simulink model "network_motif_controller_linear"  (R2022b)
settings: Solver=VariableStepAuto  StartTime=0.0  StopTime=120  RelTol=1e-3
settings Model: Creator=u1473578  LastModifiedBy=u1473578
settings DebuggingCC: UnconnectedInputMsg=warning  UnconnectedOutputMsg=warning  UnconnectedLineMsg=warning
settings ModelReferenceCC: EnableRefExpFcnMdlSchedulingChecks=on
settings RTWCC: DLArmComputeVersion=19.05

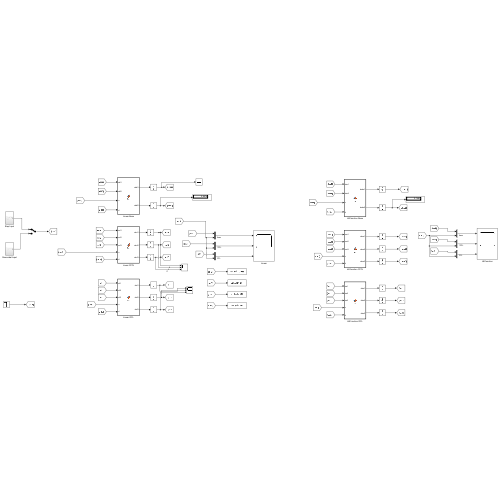
[thumbnail: Simulink's stored preview of the top-level diagram]
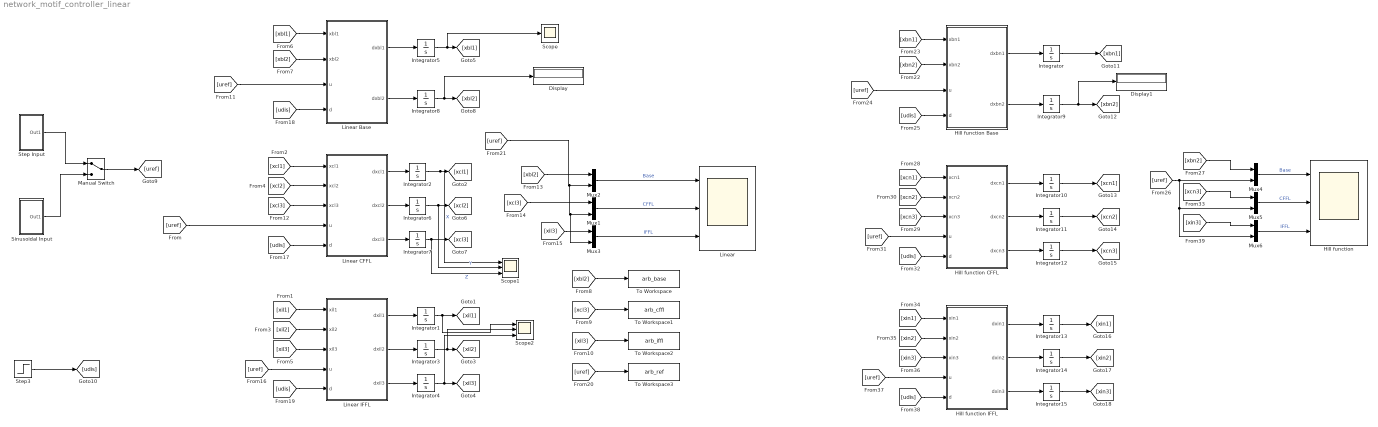
== system network_motif_controller_linear ==
  Display : Display
  Display1 : Display
  Hill function : Scope  NumInputPorts=3
  Hill function Base : MATLAB Function  TreatAsAtomicUnit=on
  Hill function CFFL : MATLAB Function  TreatAsAtomicUnit=on
  Hill function IFFL : MATLAB Function  TreatAsAtomicUnit=on
  Integrator{,1..15} (16 alike) : Integrator
  Linear : Scope  NumInputPorts=3
  Linear Base : MATLAB Function  TreatAsAtomicUnit=on
  Linear CFFL : MATLAB Function  TreatAsAtomicUnit=on
  Linear IFFL : MATLAB Function  TreatAsAtomicUnit=on
  Manual Switch : ManualSwitch
  Mux{1..6} (6 alike) : Mux  Inputs=2
  Scope : Scope
  Scope1 : Scope  NumInputPorts=3
  Scope2 : Scope  NumInputPorts=3
  Sinusoidal Input : Subsystem
  Step Input : Subsystem
  Step3 : Step  Time=60  After=-0.25*1  SampleTime=0
  To Workspace : ToWorkspace  VariableName=arb_base  SaveFormat=Timeseries  SampleTime=-1
  To Workspace1 : ToWorkspace  VariableName=arb_cffl  SaveFormat=Timeseries  SampleTime=-1
  To Workspace2 : ToWorkspace  VariableName=arb_iffl  SaveFormat=Timeseries  SampleTime=-1
  To Workspace3 : ToWorkspace  VariableName=arb_ref  SaveFormat=Timeseries  SampleTime=-1
  wires:
  Integrator2/1 -> Scope1/1, [xcl1]  "X"
  Linear CFFL/3(dxcl3) -> Integrator7/1
  [xil3] -> Mux3/1
  [xcl1] -> Linear CFFL/1(xcl1)
  Integrator7/1 -> Scope1/3, [xcl3]  "Z"
  [xcl2] -> Linear CFFL/2(xcl2)
  Mux3/1 -> Linear/3  "IFFL"
  [xcl3] -> Linear CFFL/3(xcl3)
  Linear CFFL/2(dxcl2) -> Integrator6/1
  Integrator6/1 -> Scope1/2, [xcl2]  "Y"
  Linear CFFL/1(dxcl1) -> Integrator2/1
  [xil1] -> Linear IFFL/1(xil1)
  [xil2] -> Linear IFFL/2(xil2)
  [xil3] -> Linear IFFL/3(xil3)
  Linear IFFL/1(dxil1) -> Integrator1/1
  Linear IFFL/2(dxil2) -> Integrator3/1
  Linear IFFL/3(dxil3) -> Integrator4/1
  Integrator1/1 -> Scope2/1, [xil1]
  Integrator3/1 -> Scope2/2, [xil2]
  Integrator4/1 -> Scope2/3, [xil3]
  [xcl3] -> Mux1/1
  Mux1/1 -> Linear/2  "CFFL"
  [xbl1] -> Linear Base/1(xbl1)
  [xbl2] -> Linear Base/2(xbl2)
  Linear Base/1(dxbl1) -> Integrator5/1
  Linear Base/2(dxbl2) -> Integrator8/1
  Integrator5/1 -> Scope/1, [xbl1]
  Integrator8/1 -> Display/1, [xbl2]
  Mux2/1 -> Linear/1  "Base"
  [xbl2] -> Mux2/1
  [xcl3] -> To Workspace1/1
  [xil3] -> To Workspace2/1
  [xbl2] -> To Workspace/1
  [uref] -> Linear CFFL/4(u)
  [uref] -> Linear Base/3(u)
  [uref] -> Linear IFFL/4(u)
  Step3/1 -> [udis]
  [udis] -> Linear CFFL/5(d)
  [udis] -> Linear Base/4(d)
  [udis] -> Linear IFFL/5(d)
  [uref] -> To Workspace3/1
  [uref] -> Mux3/2, Mux1/2, Mux2/2
  Hill function Base/1(dxbn1) -> Integrator/1
  Hill function Base/2(dxbn2) -> Integrator9/1
  Integrator/1 -> [xbn1]
  Integrator9/1 -> Display1/1, [xbn2]
  [xbn2] -> Hill function Base/2(xbn2)
  [xbn1] -> Hill function Base/1(xbn1)
  [uref] -> Hill function Base/3(u)
  [udis] -> Hill function Base/4(d)
  [uref] -> Mux6/2, Mux5/2, Mux4/2
  [xbn2] -> Mux4/1
  Mux4/1 -> Hill function/1  "Base"
  Hill function CFFL/1(dxcn1) -> Integrator10/1
  Hill function CFFL/2(dxcn2) -> Integrator11/1
  Hill function CFFL/3(dxcn3) -> Integrator12/1
  Integrator10/1 -> [xcn1]
  Integrator11/1 -> [xcn2]
  Integrator12/1 -> [xcn3]
  [xcn3] -> Hill function CFFL/3(xcn3)
  [xcn2] -> Hill function CFFL/2(xcn2)
  [xcn1] -> Hill function CFFL/1(xcn1)
  [uref] -> Hill function CFFL/4(u)
  [udis] -> Hill function CFFL/5(d)
  Mux5/1 -> Hill function/2  "CFFL"
  [xcn3] -> Mux5/1
  Hill function IFFL/1(dxin1) -> Integrator13/1
  Hill function IFFL/2(dxin2) -> Integrator14/1
  Hill function IFFL/3(dxin3) -> Integrator15/1
  Integrator13/1 -> [xin1]
  Integrator14/1 -> [xin2]
  Integrator15/1 -> [xin3]
  [xin1] -> Hill function IFFL/1(xin1)
  [xin2] -> Hill function IFFL/2(xin2)
  [xin3] -> Hill function IFFL/3(xin3)
  [uref] -> Hill function IFFL/4(u)
  [udis] -> Hill function IFFL/5(d)
  Mux6/1 -> Hill function/3  "IFFL"
  [xin3] -> Mux6/1
  Step Input/1(Out1) -> Manual Switch/1
  Sinusoidal Input/1(Out1) -> Manual Switch/2
  Manual Switch/1 -> [uref]

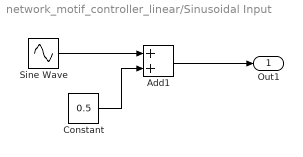
== system network_motif_controller_linear/Sinusoidal Input ==
  Add1 : Sum
  Constant : Constant  Value=0.5
  Sine Wave : Sin  Amplitude=0.5  Frequency=10/120  Phase=2800-150  SampleTime=0
  Out1 : Outport
  wires:
  Sine Wave/1 -> Add1/1
  Constant/1 -> Add1/2
  Add1/1 -> Out1/1

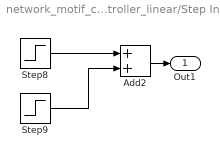
== system network_motif_controller_linear/Step Input ==
  Add2 : Sum
  Step8 : Step  Time=0  After=0  SampleTime=0
  Step9 : Step  Time=40  SampleTime=0
  Out1 : Outport
  wires:
  Step8/1 -> Add2/1
  Step9/1 -> Add2/2
  Add2/1 -> Out1/1

== matlab function network_motif_controller_linear/Linear IFFL ==
  data: xil1 input; xil2 input; xil3 input; u input; dxil1 output; dxil2 output; d input; dxil3 output
function [dxil1,dxil2,dxil3] = fcn(xil1,xil2,xil3,u,d)

% x1 = X
% x2 = Y
% x3 = Z
c = 1*1;
gamma = 1;
delta_x = 0.01*1;

alpha_y = 1;
delta_y = 10*1;

alpha_z1 = 1;
alpha_z2 = 1;
delta_z = 1;

dxil1 = c*u - gamma*xil3 - delta_x*xil1;

dxil2 = alpha_y*xil1 - delta_y*xil2;

dxil3 = alpha_z1*xil1 - alpha_z2*xil2 - delta_z*xil3 + d;

== matlab function network_motif_controller_linear/Linear Base ==
  data: xbl1 input; xbl2 input; u input; dxbl1 output; dxbl2 output; d input
function [dxbl1,dxbl2] = fcn(xbl1,xbl2,u,d)

% x1 = X
% x2 = Z

% gamma = 1;
% delta_x = 0.01;
% alpha_z = 0.002;
% delta_z = 0.004;
% alpha_d = 0.05;

% gamma = 1;
% delta_x = 0.01;
% alpha_z = 1;
% delta_z = 0.004;
% alpha_d = 0.05;

% Arbitrary Parameters
gamma = 1;
c = 1*1;
delta_x = 0.01 * 1;
alpha_z = 1;
delta_z = 1;
alpha_d = 1;

dxbl1 = c*u - gamma*xbl2 - delta_x*xbl1;

dxbl2 = alpha_z*xbl1 - delta_z*xbl2 + alpha_d*d;

== matlab function network_motif_controller_linear/Hill function Base ==
  data: xbn1 input; xbn2 input; u input; dxbn1 output; dxbn2 output; d input
function [dxbn1,dxbn2] = fcn(xbn1,xbn2,u,d)

% x1 = X
% x2 = Z

gamma = 1;
c = gamma;
%% Derived Parameters through two-point matching (Inhibition Type 1)
% Kx = 0.002;
% Kz = 0.08;
% 
% % per minutes
% delta_x = 0.0005;
% delta_z = 0.02;
% 
% alpha_x = 2e-8;
% alpha_z = 1e-4;
% 
% bs = -5e-3;

%% Derived Parameters through two-point matching (Inhibition Type 2)
Kx = 0.4;
Kz = 0.4;

% per minutes
delta_x = 0.01;
delta_z = 1;

alpha_x = 1.;
alpha_z = 1;

bs = -1.0;


%% Matthew's Parameters (Inhibiition Type 2)
% Kx = sqrt(0.05);
% Kz = sqrt(0.05);
% 
% % per minutes
% delta_x = 0.5;
% delta_z = 0.5;
% 
% alpha_x = 0.5;
% alpha_z = 0.5;
% 
% bs = -0.5;

%% ODE

% Inhibition Type 1
% dxbn1 = c*u + ((alpha_x)/(Kx^2 + xbn2^2) + bs) - delta_x*xbn1;

% Inhibition Type 2
dxbn1 = c*u + ((alpha_x*Kx^2)/(Kx^2 + xbn2^2) + bs) - delta_x*xbn1;

dxbn2 = (alpha_z*xbn1^2/(Kz^2 + xbn1^2)) - delta_z*xbn2 + 1*d;

== matlab function network_motif_controller_linear/Linear CFFL ==
  data: xcl1 input; xcl2 input; xcl3 input; u input; dxcl1 output; dxcl2 output; d input; dxcl3 output
function [dxcl1,dxcl2,dxcl3] = fcn(xcl1,xcl2,xcl3,u,d)

% x1 = X
% x2 = Y
% x3 = Z
c = 1*1;
gamma = 1;
delta_x = 0.01 * 1;

alpha_y = 1;
delta_y = 10*1;

alpha_z1 = 1;
alpha_z2 = 1*1;
delta_z = 1;

dxcl1 = c*u - gamma*xcl3 - delta_x*xcl1;

dxcl2 = alpha_y*xcl1 - delta_y*xcl2;

dxcl3 = alpha_z1*xcl1 + alpha_z2*xcl2 - delta_z*xcl3 + d;

== matlab function network_motif_controller_linear/Hill function CFFL ==
  data: xcn1 input; xcn2 input; xcn3 input; u input; dxcn1 output; dxcn2 output; d input; dxcn3 output
function [dxcn1,dxcn2,dxcn3] = fcn(xcn1,xcn2,xcn3,u,d)

gamma = 1;
c = gamma;

Kx = 0.4;
Ky = 0.4; 
Kz1 = 0.4; 
Kz2 = 0.04*10; 

delta_x = 0.01;
delta_y = 10;
delta_z = 1;

alpha_x = 1;
alpha_y = 1; 
alpha_z1 = 1; 
alpha_z2 = 0.1*10; 

bs = -1;



dxcn1 = c*u + ((alpha_x*Kx^2)/(Kx^2 + xcn3^2) + bs) - delta_x*xcn1;

dxcn2 = (alpha_y*xcn1^2)/(Ky^2 + xcn1^2) - delta_y*xcn2;

dxcn3 = (alpha_z1*xcn1^2/(Kz1^2 + xcn1^2)) + (alpha_z2*xcn2^2/(Kz2^2 + xcn2^2)) - delta_z*xcn3 + 1*d;

== matlab function network_motif_controller_linear/Hill function IFFL ==
  data: xin1 input; xin2 input; xin3 input; u input; dxin1 output; dxin2 output; d input; dxin3 output
function [dxin1,dxin2,dxin3] = fcn(xin1,xin2,xin3,u,d)

gamma = 1;
c = gamma;

% 1.0331    1.0331    2.9465    0.4144

Kx = 0.4;
Ky = 0.4; 
% Kz1 = 0.4; 
% Kz2 = 0.04; 

% Kz1 = 4.4363-2.4;
% Kz2 = 0.4019+0.1;

Kz1 = 2.9465;
Kz2 = 0.4144;

delta_x = 0.01;
delta_y = 10;
delta_z = 1;

alpha_x = 1;
alpha_y = 1; 
% alpha_z1 = 1; 
% alpha_z2 = 0.1; 

alpha_z1 = 1.5624*1.3;
alpha_z2 = 1.5624*1.3;

% alpha_z1 = 1.0331;
% alpha_z2 = 1.0331;


bs = -1;
bsz = -0.1;

%% Matthew's Parameters (Inhibiition Type 2)
% Kx = 0.05;
% Kz = 0.05;
% 
% % per minutes
% delta_x = 0.5;
% delta_z = 0.5;
% 
% alpha_x = 0.5;
% alpha_z = 0.5;
% 
% bs = -0.5;

%% ODE


% Inhibition Type 2
dxin1 = c*u + ((alpha_x*Kx^2)/(Kx^2 + xin3^2) + bs) - delta_x*xin1;

dxin2 = (alpha_y*xin1^2)/(Ky^2 + xin1^2) - delta_y*xin2;

% dxin3 = (alpha_z1*xin1^2/(Kz1^2 + xin1^2)) + (alpha_z2*Kz2^2/(Kz2^2 + xin2^2) + bsz) - delta_z*xin3 + 1*d; % 2-term
dxin3 = (alpha_z1*xin1^2/(Kz1^2 + xin1^2)) * (alpha_z2*Kz2^2/(Kz2^2 + xin2^2)) - delta_z*xin3 + 1*d; % 2-term
